simulink model "IntModelY1"  (R2022b)
settings: Solver=VariableStepAuto  StartTime=0.0  StopTime=inf  RelTol=1e-3
model workspace (MAT data in the model file):
  firstWarning = 1
  originalScenarioChecksum = '114339432DE22364D47BB28FC96DC10C'
undefined symbols (not defined in the file): Acceleration, ActorID, AngularVelocity, curvature, curvatureAhd, DefaultGear, DEND_B, DEND_S, DEND_T, direction, driving, gradbp, L, LF, LR, matlabshared, MAX_BRAKE, MAX_STEER, MAX_TORQUE, MCAR, MIN_BRAKE, MIN_STEER, MIN_TORQUE, NUMD_B, NUMD_S, NUMD_T, Pitch, Position, psi_o, R, Roll, RRdamp, SceneInfo, session, sigbuilder_block, STEER_RATIO, stopSign_ID, Tdead, thetaRefs, TL_ID, TrackWidth, Ts, ts, Vdead, Velocity, WB, X_o, xRef2s, Y_o, Yaw, yRef2s
libraries: drivingscenarioandsensors x8, simulink x4, drivingvehiclecontroller x2, trackingutilitieslib x2, simulink_extras x2, robotalgslib x1, mpcadaslib x1, drivinglib x1, autolibshared x1, vehdynlibviscommon x1, vehdynlibsteering x1
(part 1 of 3)
settings Model: Creator=akshran  LastModifiedBy=deepikagiridhar
settings DataIOCC: SignalLogging=off
settings DebuggingCC: UnconnectedInputMsg=warning  UnconnectedOutputMsg=warning  UnconnectedLineMsg=warning
settings ModelReferenceCC: EnableRefExpFcnMdlSchedulingChecks=on
settings RTWCC: DLArmComputeVersion=19.05

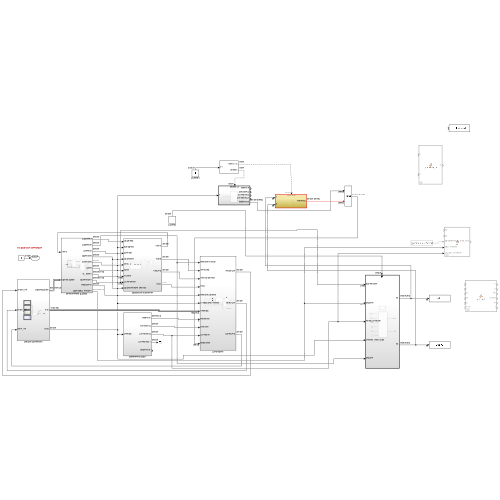
[thumbnail: Simulink's stored preview of the top-level diagram]
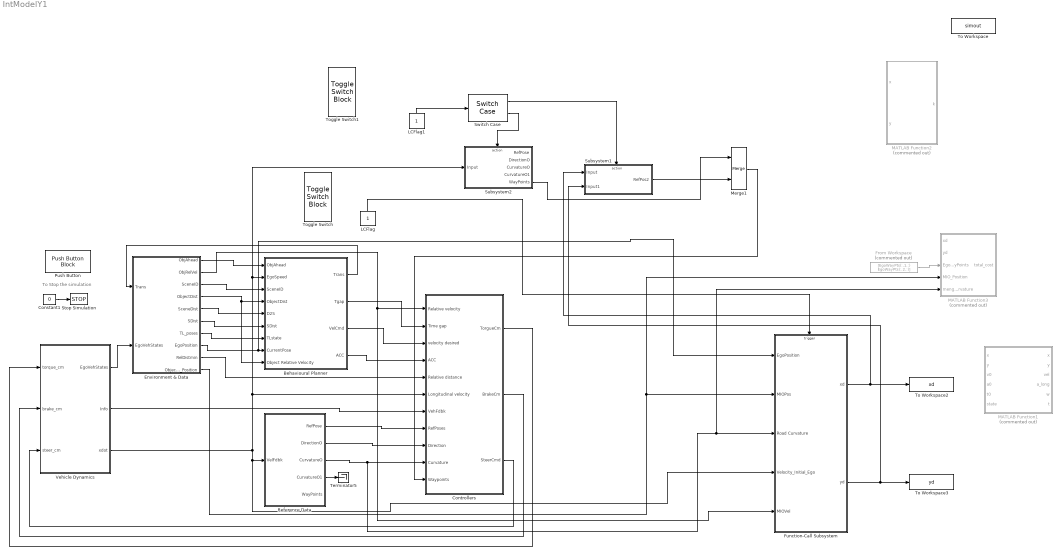
== system IntModelY1 ==
  note: To Stop the simulation
  Behavioural Planner : Subsystem
  Constant1 : Constant  Value=0
  Controllers : Subsystem
  Environment & Data : Subsystem
  From Workspace : FromWorkspace  Commented=on  VariableName=[EgoWayPts(:,1,:) EgoWayPts(:,2,:)]
  Function-Call Subsystem : Subsystem  TreatAsAtomicUnit=on
  LCFlag : Constant
  LCFlag1 : Constant
  MATLAB Function1 : MATLAB Function  Commented=on  TreatAsAtomicUnit=on
  MATLAB Function2 : MATLAB Function  Commented=on  TreatAsAtomicUnit=on
  MATLAB Function3 : MATLAB Function  Commented=on  TreatAsAtomicUnit=on
  Merge1 : Merge
  Push Button : PushButtonBlock  OffValue=1.000000
  Reference Data : Subsystem  VariantControl=Stanley
  Stop Simulation : Stop
  Subsystem1 : Subsystem
  Subsystem2 : Subsystem
  Switch Case : SwitchCase
  Terminator5 : Terminator
  To Workspace : ToWorkspace  VariableName=simout  SaveFormat=Timeseries  SampleTime=-1
  To Workspace2 : ToWorkspace  VariableName=xd  SaveFormat=Timeseries  SampleTime=-1
  To Workspace3 : ToWorkspace  VariableName=yd  SaveFormat=Timeseries  SampleTime=-1
  Toggle Switch : ToggleSwitchBlock
      settings: Values={{'Off', 'On'}, [0 1]}
  Toggle Switch1 : ToggleSwitchBlock
      settings: Values={{'Off', 'On'}, [0 1]}
  Vehicle Dynamics : Subsystem
  wires:
  Environment & Data/4(ObjectDist) -> Behavioural Planner/9(Object Relative Velocity), Behavioural Planner/4(ObjectDist)
  Environment & Data/2(ObjRelVel) -> Function-Call Subsystem/5(MIOVel), Controllers/1(Relative velocity)
  Environment & Data/8(EgoPosition) -> Function-Call Subsystem/1(EgoPosition), Behavioural Planner/8(CurrentPose)
  Vehicle Dynamics/1(EgoVehStates) -> Environment & Data/2(EgoVehStates)
  Vehicle Dynamics/2(Info) -> Controllers/7(VehFdbk)
  Environment & Data/5(SceneDist) -> Behavioural Planner/5(D2S)
  Environment & Data/3(SceneID) -> Behavioural Planner/3(SceneID)
  Behavioural Planner/4(ACC) -> Controllers/4(ACC)
  Environment & Data/9(RelDistmin) -> Controllers/5(Relative distance)
  Environment & Data/1(ObjAhead) -> Behavioural Planner/1(ObjAhead)
  Vehicle Dynamics/3(xdot) -> Subsystem2/1(Input), Behavioural Planner/2(EgoSpeed), Controllers/6(Longitudinal velocity), Function-Call Subsystem/4(Velocity_Initial_Ego), Reference Data/1(VelFdbk)
  Environment & Data/6(SDist) -> Behavioural Planner/6(SDist)
  Environment & Data/7(TL_poses) -> Behavioural Planner/7(TLstate)
  Controllers/2(BrakeCm) -> Vehicle Dynamics/2(brake_cm)
  Behavioural Planner/1(Trans) -> Environment & Data/1(Trans)
  Behavioural Planner/2(Tgap) -> Controllers/2(Time gap)
  Behavioural Planner/3(VelCmd) -> Controllers/3(velocity desired)
  Reference Data/2(DirectionO) -> Controllers/9(Direction)
  Reference Data/3(CurvatureO) -> Function-Call Subsystem/3(Road Curvature), MATLAB Function3/5(menger_curvature), Controllers/10(Curvature)
  Reference Data/4(CurvatureO1) -> Terminator5/1
  Controllers/1(TorgueCm) -> Vehicle Dynamics/1(torque_cm)
  Controllers/3(SteerCmd) -> Vehicle Dynamics/3(steer_cm)
  Constant1/1 -> Stop Simulation/1
  From Workspace/1 -> MATLAB Function3/3(EgoWayPoints)
  Environment & Data/10(ObjectMIO_Position) -> MATLAB Function3/4(MIO_Position), Function-Call Subsystem/2(MIOPos)
  LCFlag/1 -> Function-Call Subsystem/Trigger
  Function-Call Subsystem/1(xd) -> Subsystem1/1(Input), To Workspace2/1
  Function-Call Subsystem/2(yd) -> Subsystem1/2(Input1), To Workspace3/1
  Switch Case/2 -> Subsystem2/Action
  Switch Case/1 -> Subsystem1/Action
  Reference Data/1(RefPose) -> Controllers/8(RefPoses)
  Subsystem2/5(WayPoints) -> Merge1/1
  Merge1/1 -> Controllers/11(Waypoints)
  LCFlag1/1 -> Switch Case/1
  Subsystem1/1(RefPos2) -> Merge1/2

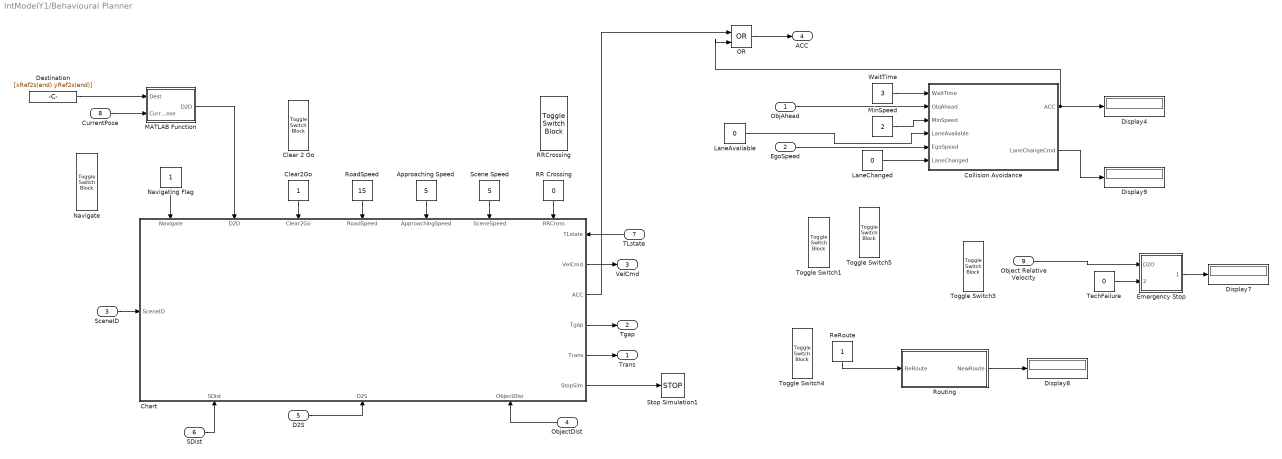
== system IntModelY1/Behavioural Planner ==
  ObjAhead : Inport
  EgoSpeed : Inport  Port=2
  SceneID : Inport  Port=3
  ObjectDist : Inport  Port=4
  D2S : Inport  Port=5
  SDist : Inport  Port=6
  TLstate : Inport  Port=7
  CurrentPose : Inport  Port=8
  Object Relative Velocity : Inport  Port=9
  Approaching Speed : Constant  Value=5
  Chart : Stateflow chart  TreatAsAtomicUnit=on
      settings: PortSchema="{\"entries\":[{\"content\":{\"sides\":[{\"content\":{\"connectorIds\":[\"In12\"]},\"type\":\"ConnectorPlacement.EquallySpacedRectSide\",\"uuid\":\"81aca70f-0947-49fb-b60a-be241e44193b\"},{\"content\":{\"connectorIds\":[\"In1\",\"Out1\",\"Out2\",\"Out3\",\"Out4\",\"Out5\"],\"side\":\"RIGHT\"},\"type\":\"ConnectorPlacement.EquallySpacedRectSide\",\"uuid\":\"e7b9645e-3711-4964-ac9b-0199dd335e99\"},{\"content\":{\"connectorIds\":[\"In8\",\"In9\",\"In10\",\"In11\",\"In2\",\"In4\",\"In6\"],\"side\":\"TOP\"},\"type\":\"ConnectorPlacement.EquallySpacedRectSide\",\"uuid\":\"6876f024-944b-4540-9404-d68f37763657\"},{\"content\":{\"connectorIds\":[\"In5\",\"In7\",\"In3\"],\"side\":\"BOTTOM\"},\"type\":\"ConnectorPlacement.EquallySpacedRectSide\",\"uuid\":\"44acab73-cdde-4edf-95df-27422644ccab\"}]},\"type\":\"ConnectorPlacement.EquallySpacedConnector\",\"uuid\":\"d2c31c01-e447-43db-8d2b-8b98a0ca291a\"}],\"packageUris\":[\"http://schema.mathworks.com/mf0/Connector/R2020b\"],\"version\":\"1.0\"}"
  Clear 2 Go : ToggleSwitchBlock
      settings: Values={{'Off', 'On'}, [0 1]}
  Clear2Go : Constant
  Collision Avoidance : Stateflow chart  TreatAsAtomicUnit=on
  Destination : Constant  Value=[xRef2s(end) yRef2s(end)]
  Display{4,7..9} (4 alike) : Display
  Emergency Stop : Stateflow chart  TreatAsAtomicUnit=on
  LaneAvailable : Constant  Value=0
  LaneChanged : Constant  Value=0
  MATLAB Function : MATLAB Function  TreatAsAtomicUnit=on
  MinSpeed : Constant  Value=2
  Navigate : ToggleSwitchBlock
      settings: Values={{'Off', 'On'}, [0 1]}
  Navigating Flag : Constant
  OR : Logic  Operator=OR  IconShape=distinctive  AllPortsSameDT=off  OutDataTypeStr=fixdt(1,16)
  RR Crossing : Constant  Value=0
  RRCrossing : ToggleSwitchBlock
      settings: Values={{'Off', 'On'}, [0 1]}
  ReRoute : Constant
  RoadSpeed : Constant  Value=15
  Routing : Stateflow chart  TreatAsAtomicUnit=on
  Scene Speed : Constant  Value=5
  Stop Simulation1 : Stop
  TechFailure : Constant  Value=0
  Toggle Switch{1,3..5} (4 alike) : ToggleSwitchBlock
      settings: Values={{'Off', 'On'}, [0 1]}
  WaitTime : Constant  Value=3
  Trans : Outport
  Tgap : Outport  Port=2
  VelCmd : Outport  Port=3
  ACC : Outport  Port=4
  wires:
  Clear2Go/1 -> Chart/10(Clear2Go)
  Routing/1(NewRoute) -> Display8/1
  ObjectDist/1 -> Chart/3(ObjectDist)
  WaitTime/1 -> Collision Avoidance/1(WaitTime)
  Navigating Flag/1 -> Chart/8(Navigate)
  Approaching Speed/1 -> Chart/2(ApproachingSpeed)
  Scene Speed/1 -> Chart/4(SceneSpeed)
  EgoSpeed/1 -> Collision Avoidance/5(EgoSpeed)
  ReRoute/1 -> Routing/1(ReRoute)
  Collision Avoidance/2(LaneChangeCmd) -> Display9/1
  LaneAvailable/1 -> Collision Avoidance/4(LaneAvailable)
  CurrentPose/1 -> MATLAB Function/2(CurrentPose)
  RR Crossing/1 -> Chart/6(RRCross)
  MinSpeed/1 -> Collision Avoidance/3(MinSpeed)
  LaneChanged/1 -> Collision Avoidance/6(LaneChanged)
  RoadSpeed/1 -> Chart/11(RoadSpeed)
  ObjAhead/1 -> Collision Avoidance/2(ObjAhead)
  Destination/1 -> MATLAB Function/1(Dest)
  SceneID/1 -> Chart/12(SceneID)
  MATLAB Function/1(D2D) -> Chart/9(D2D)
  Chart/5(StopSim) -> Stop Simulation1/1
  Chart/4(Trans) -> Trans/1
  TLstate/1 -> Chart/1(TLstate)
  Chart/1(VelCmd) -> VelCmd/1
  SDist/1 -> Chart/5(SDist)
  D2S/1 -> Chart/7(D2S)
  Chart/3(Tgap) -> Tgap/1
  TechFailure/1 -> Emergency Stop/2(TechFailure)
  Emergency Stop/1(EStop) -> Display7/1
  Object Relative Velocity/1 -> Emergency Stop/1(D2O)
  Collision Avoidance/1(ACC) -> OR/2, Display4/1
  OR/1 -> ACC/1
  Chart/2(ACC) -> OR/1

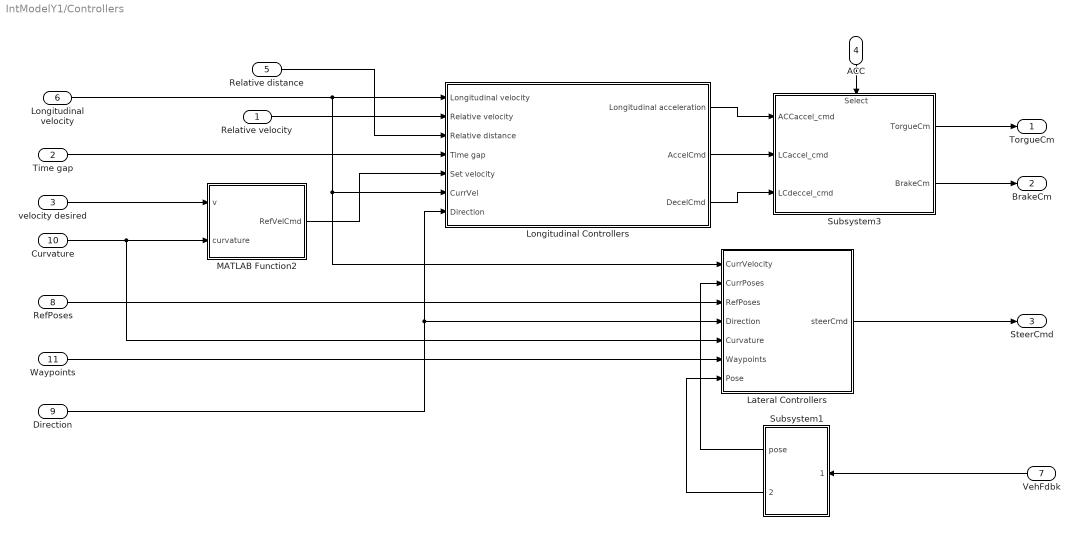
== system IntModelY1/Controllers ==
  Relative velocity : Inport
  Time gap : Inport  Port=2
  velocity desired : Inport  Port=3
  ACC : Inport  Port=4
  Relative distance : Inport  Port=5
  Longitudinal velocity : Inport  Port=6
  VehFdbk : Inport  Port=7
  RefPoses : Inport  Port=8
  Direction : Inport  Port=9
  Curvature : Inport  Port=10
  Waypoints : Inport  Port=11
  Lateral Controllers : Subsystem
  Longitudinal Controllers : Subsystem
  MATLAB Function2 : MATLAB Function  TreatAsAtomicUnit=on
  Subsystem1 : Subsystem
  Subsystem3 : Subsystem
      settings: PortSchema="{\"entries\":[{\"content\":{\"sides\":[{\"content\":{\"connectorIds\":[\"In1\",\"In2\",\"In3\"]},\"type\":\"ConnectorPlacement.EquallySpacedRectSide\",\"uuid\":\"a23b1a10-3bcb-40a0-900c-c9a3f160b173\"},{\"content\":{\"connectorIds\":[\"Out1\",\"Out2\"],\"side\":\"RIGHT\"},\"type\":\"ConnectorPlacement.EquallySpacedRectSide\",\"uuid\":\"88840b66-912f-4184-aeec-297642319416\"},{\"content\":{\"connectorIds\":[\"In4\"],\"side\":\"TOP\"},\"type\":\"ConnectorPlacement.EquallySpacedRectSide\",\"uuid\":\"37a03ca9-b065-473e-b290-3b07703c6005\"}]},\"type\":\"ConnectorPlacement.EquallySpacedConnector\",\"uuid\":\"5bfc7c71-8f7a-4cba-a168-7eeca22a2fcb\"}],\"packageUris\":[\"http://schema.mathworks.com/mf0/Connector/R2020b\"],\"version\":\"1.0\"}"
  TorgueCm : Outport
  BrakeCm : Outport  Port=2
  SteerCmd : Outport  Port=3
  wires:
  Subsystem1/1(pose) -> Lateral Controllers/2(CurrPoses)
  Longitudinal Controllers/1(Longitudinal acceleration) -> Subsystem3/1(ACCaccel_cmd)
  Curvature/1 -> Lateral Controllers/5(Curvature), MATLAB Function2/2(curvature)
  Relative velocity/1 -> Longitudinal Controllers/2(Relative velocity)
  Subsystem1/2(PPpose) -> Lateral Controllers/7(Pose)
  MATLAB Function2/1(RefVelCmd) -> Longitudinal Controllers/5(Set velocity)
  Direction/1 -> Lateral Controllers/4(Direction), Longitudinal Controllers/7(Direction)
  RefPoses/1 -> Lateral Controllers/3(RefPoses)
  velocity desired/1 -> MATLAB Function2/1(v)
  Subsystem3/2(BrakeCm) -> BrakeCm/1
  Longitudinal Controllers/2(AccelCmd) -> Subsystem3/2(LCaccel_cmd)
  Longitudinal Controllers/3(DecelCmd) -> Subsystem3/3(LCdeccel_cmd)
  Longitudinal velocity/1 -> Lateral Controllers/1(CurrVelocity), Longitudinal Controllers/6(CurrVel), Longitudinal Controllers/1(Longitudinal velocity)
  Time gap/1 -> Longitudinal Controllers/4(Time gap)
  Waypoints/1 -> Lateral Controllers/6(Waypoints)
  VehFdbk/1 -> Subsystem1/1(VehFdbk)
  Subsystem3/1(TorgueCm) -> TorgueCm/1
  Lateral Controllers/1(steerCmd) -> SteerCmd/1
  Relative distance/1 -> Longitudinal Controllers/3(Relative distance)
  ACC/1 -> Subsystem3/4(Select)

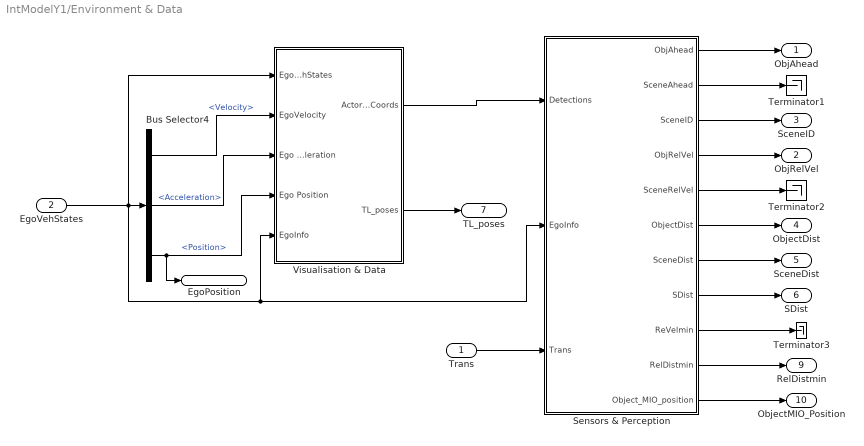
== system IntModelY1/Environment & Data ==
  Trans : Inport
  EgoVehStates : Inport  Port=2
  Bus Selector4 : BusSelector  OutputSignals=Velocity,Acceleration,Position
  Sensors & Perception : Subsystem
  Terminator1 : Terminator
  Terminator2 : Terminator
  Terminator3 : Terminator
  Visualisation & Data : Subsystem
  ObjAhead : Outport
  ObjRelVel : Outport  Port=2
  SceneID : Outport  Port=3
  ObjectDist : Outport  Port=4
  SceneDist : Outport  Port=5
  SDist : Outport  Port=6
  TL_poses : Outport  Port=7
  EgoPosition : Outport  Port=8
  RelDistmin : Outport  Port=9
  ObjectMIO_Position : Outport  Port=10
  wires:
  EgoVehStates/1 -> Visualisation & Data/1(EgoVehStates), Sensors & Perception/2(EgoInfo), Visualisation & Data/5(EgoInfo), Bus Selector4/1
  Bus Selector4/2 -> Visualisation & Data/3(Ego Acceleration)  "<Acceleration>"
  Bus Selector4/1 -> Visualisation & Data/2(EgoVelocity)  "<Velocity>"
  Visualisation & Data/2(TL_poses) -> TL_poses/1
  Sensors & Perception/1(ObjAhead) -> ObjAhead/1
  Sensors & Perception/7(SceneDist) -> SceneDist/1
  Bus Selector4/3 -> Visualisation & Data/4(Ego Position), EgoPosition/1  "<Position>"
  Visualisation & Data/1(Actors_VehCoords) -> Sensors & Perception/1(Detections)
  Trans/1 -> Sensors & Perception/3(Trans)
  Sensors & Perception/2(SceneAhead) -> Terminator1/1
  Sensors & Perception/3(SceneID) -> SceneID/1
  Sensors & Perception/4(ObjRelVel) -> ObjRelVel/1
  Sensors & Perception/5(SceneRelVel) -> Terminator2/1
  Sensors & Perception/6(ObjectDist) -> ObjectDist/1
  Sensors & Perception/8(SDist) -> SDist/1
  Sensors & Perception/9(ReVelmin) -> Terminator3/1
  Sensors & Perception/10(RelDistmin) -> RelDistmin/1
  Sensors & Perception/11(Object_MIO_position) -> ObjectMIO_Position/1

== system IntModelY1/Function-Call Subsystem ==
  EgoPosition : Inport
  MIOPos : Inport  Port=2
  Road Curvature : Inport  Port=3
  Velocity_Initial_Ego : Inport  Port=4
  MIOVel : Inport  Port=5
  function : TriggerPort  VariantControl=(inherit)  ShowOutputPort=on
  Constant : Constant
  MATLAB Function : MATLAB Function  TreatAsAtomicUnit=on
  xd : Outport
  yd : Outport  Port=2
  wires:
  EgoPosition/1 -> MATLAB Function/1(EgoPosition)
  MIOPos/1 -> MATLAB Function/2(MIOPos)
  Road Curvature/1 -> MATLAB Function/3(curvature)
  MIOVel/1 -> MATLAB Function/4(MIOVel)
  Velocity_Initial_Ego/1 -> MATLAB Function/5(V_i)
  MATLAB Function/1(xd) -> xd/1
  MATLAB Function/2(yd) -> yd/1
  Constant/1 -> MATLAB Function/6(lane_side)

== system IntModelY1/Reference Data ==
  note: Select method to calculate theta
  VelFdbk : Inport
  Curvature : Lookup_n-D  NumberOfTableDimensions=1  BreakpointsForDimension1=gradbp  Table=curvature  InternalRulePriority=Speed  RndMeth=Simplest
  CurvatureAhd : Lookup_n-D  Commented=on  NumberOfTableDimensions=1  BreakpointsForDimension1=gradbp  Table=curvatureAhd  InternalRulePriority=Speed  RndMeth=Simplest
  Direction : Lookup_n-D  NumberOfTableDimensions=1  BreakpointsForDimension1=gradbp  Table=direction  InternalRulePriority=Speed  RndMeth=Simplest
  Integrator : Integrator
  Matrix Concatenate : Concatenate  Mode=Multidimensional array  ConcatenateDimension=2
  Mux : Mux  Inputs=3
  Theta : Subsystem  Variant=on  VariantControlMode=label  LabelModeActiveChoice=thetaLookUpTable
  X Ref : Lookup_n-D  NumberOfTableDimensions=1  BreakpointsForDimension1=gradbp  Table=xRef2s  InternalRulePriority=Speed  RndMeth=Simplest
  Y Ref : Lookup_n-D  NumberOfTableDimensions=1  BreakpointsForDimension1=gradbp  Table=yRef2s  InternalRulePriority=Speed  RndMeth=Simplest
  RefPose : Outport
  DirectionO : Outport  Port=2
  CurvatureO : Outport  Port=3
  CurvatureO1 : Outport  Port=4
  WayPoints : Outport  Port=5
  wires:
  Direction/1 -> DirectionO/1
  Curvature/1 -> CurvatureO/1
  Mux/1 -> RefPose/1
  Integrator/1 -> CurvatureAhd/1, Curvature/1, Direction/1, Matrix Concatenate/1, Theta/3(dis), Y Ref/1, Matrix Concatenate/2, X Ref/1
  VelFdbk/1 -> Integrator/1
  Theta/1(theta) -> Mux/3
  CurvatureAhd/1 -> CurvatureO1/1
  Matrix Concatenate/1 -> WayPoints/1
  X Ref/1 -> Theta/2(x), Mux/1
  Y Ref/1 -> Theta/1(y), Mux/2

== system IntModelY1/Subsystem1 ==
  Input : Inport
  Input1 : Inport  Port=2
  Action Port : ActionPort  ActionPortLabel=case [ 1 ]:
  From Workspace : FromWorkspace  Commented=on  VariableName=xRef2
  From Workspace1 : FromWorkspace  Commented=on  VariableName=yRef2
  Matrix Concatenate : Concatenate  Mode=Multidimensional array  ConcatenateDimension=2
  RefPos2 : Outport
  wires:
  Matrix Concatenate/1 -> RefPos2/1
  Input/1 -> Matrix Concatenate/1
  Input1/1 -> Matrix Concatenate/2

== system IntModelY1/Subsystem2 ==
  Input : Inport
  Action Port : ActionPort  ActionPortLabel=default:
  Reference Data : Subsystem  VariantControl=Stanley
  RefPose : Outport
  DirectionO : Outport  Port=2
  CurvatureO : Outport  Port=3
  CurvatureO1 : Outport  Port=4
  WayPoints : Outport  Port=5
  wires:
  Input/1 -> Reference Data/1(VelFdbk)
  Reference Data/1(RefPose) -> RefPose/1
  Reference Data/5(WayPoints) -> WayPoints/1
  Reference Data/4(CurvatureO1) -> CurvatureO1/1
  Reference Data/3(CurvatureO) -> CurvatureO/1
  Reference Data/2(DirectionO) -> DirectionO/1

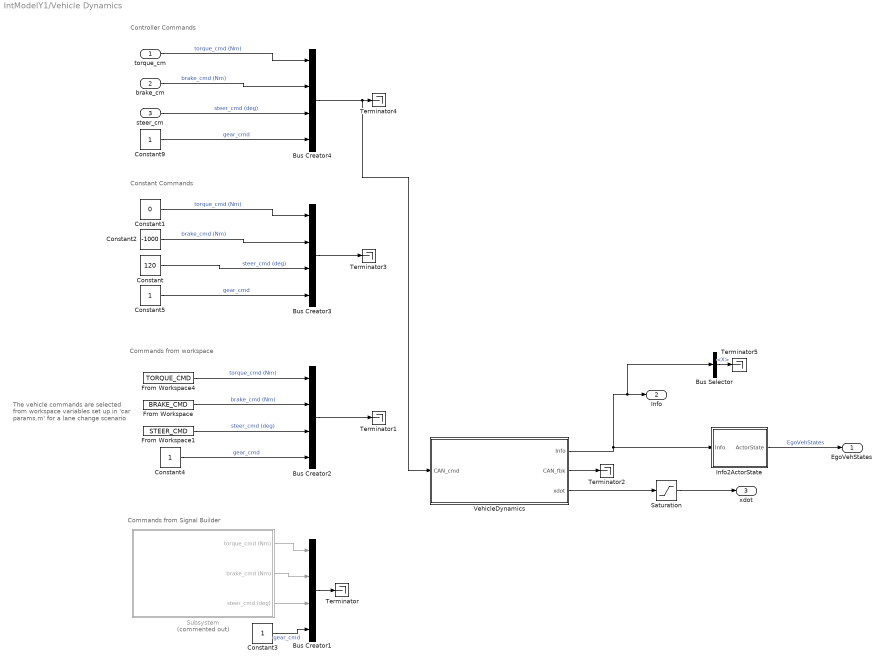
== system IntModelY1/Vehicle Dynamics ==
  note: Constant Commands
  note: Commands from workspace
  note: Commands from Signal Builder
  note: The vehicle commands are selected from workspace variables set up in 'car params.m' for a lane change scenario
  note: Controller Commands
  torque_cm : Inport
  brake_cm : Inport  Port=2
  steer_cm : Inport  Port=3
  Bus Creator{1..4} (4 alike) : BusCreator  Inputs=4
  Bus Selector : BusSelector  OutputSignals=InertFrm.Cg.Disp.X
  Constant : Constant  Value=120
  Constant1 : Constant  Value=0
  Constant2 : Constant  Value=-1000
  Constant{3..5,9} (4 alike) : Constant
  From Workspace : FromWorkspace  VariableName=BRAKE_CMD  SampleTime=ts
  From Workspace1 : FromWorkspace  VariableName=STEER_CMD  SampleTime=ts
  From Workspace4 : FromWorkspace  VariableName=TORQUE_CMD  SampleTime=ts
  Info2ActorState : Subsystem
  Saturation : Saturate  UpperLimit=inf  LowerLimit=0.001
  Subsystem : Subsystem  Commented=on
  Terminator{,1..5} (6 alike) : Terminator
  VehicleDynamics : Subsystem  mask{InitPosition=[X_o Y_o 0], InitSpeed=0, InitYaw=psi_o}
      mask prompts: InitPosition "Initial Position (m)"; InitSpeed "Initial Speed (m/s)"; InitYaw "Init Yaw (rad)"
  EgoVehStates : Outport
  Info : Outport  Port=2
  xdot : Outport  Port=3
  wires:
  Bus Creator2/1 -> Terminator1/1
  VehicleDynamics/2(CAN_fbk) -> Terminator2/1
  VehicleDynamics/1(Info) -> Bus Selector/1, Info/1, Info2ActorState/1(Info)
  Constant/1 -> Bus Creator3/3  "steer_cmd (deg)"
  Info2ActorState/1(ActorState) -> EgoVehStates/1  "EgoVehStates"
  Constant1/1 -> Bus Creator3/1  "torque_cmd (Nm)"
  Constant2/1 -> Bus Creator3/2  "brake_cmd (Nm)"
  VehicleDynamics/3(xdot) -> Saturation/1
  Subsystem/1(torque_cmd (Nm)) -> Bus Creator1/1
  Subsystem/2(brake_cmd (Nm)) -> Bus Creator1/2
  Subsystem/3(steer_cmd (deg)) -> Bus Creator1/3
  Constant3/1 -> Bus Creator1/4  "gear_cmd"
  Constant4/1 -> Bus Creator2/4  "gear_cmd"
  From Workspace/1 -> Bus Creator2/2  "brake_cmd (Nm)"
  From Workspace1/1 -> Bus Creator2/3  "steer_cmd (deg)"
  From Workspace4/1 -> Bus Creator2/1  "torque_cmd (Nm)"
  Constant5/1 -> Bus Creator3/4  "gear_cmd"
  Bus Creator1/1 -> Terminator/1
  brake_cm/1 -> Bus Creator4/2  "brake_cmd (Nm)"
  Constant9/1 -> Bus Creator4/4  "gear_cmd"
  torque_cm/1 -> Bus Creator4/1  "torque_cmd (Nm)"
  steer_cm/1 -> Bus Creator4/3  "steer_cmd (deg)"
  Bus Creator3/1 -> Terminator3/1
  Bus Creator4/1 -> VehicleDynamics/1(CAN_cmd), Terminator4/1
  Saturation/1 -> xdot/1
  Bus Selector/1 -> Terminator5/1  "<X>"

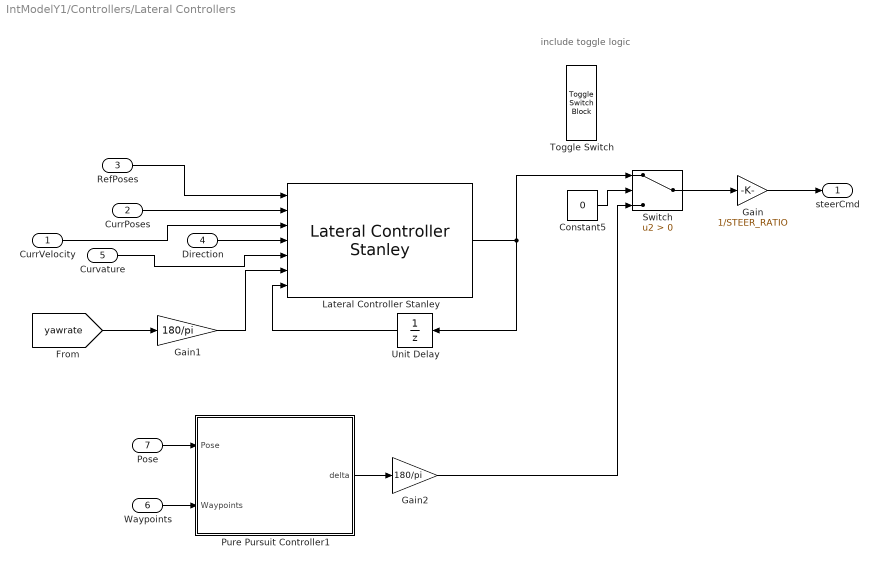
== system IntModelY1/Controllers/Lateral Controllers ==
  note: include toggle logic
  CurrVelocity : Inport
  CurrPoses : Inport  Port=2
  RefPoses : Inport  Port=3
  Direction : Inport  Port=4
  Curvature : Inport  Port=5
  Waypoints : Inport  Port=6
  Pose : Inport  Port=7
  Constant5 : Constant  Value=0
  Gain : Gain  Gain=1/STEER_RATIO
  Gain1 : Gain  Gain=180/pi
  Gain2 : Gain  Gain=180/pi
  Lateral Controller Stanley : drivingvehiclecontroller/Lateral Controller Stanley  ModelType=Dynamic bicycle model  PositionGainF=2.5  PositionGainR=2.5  YawRateGain=0.2  DelayGain=0.2  VehicleMass=MCAR  Lf=LF  Lr=LR  TireStiffness=5e3  Wheelbase=3  MaxSteeringAngle=80
  Pure Pursuit Controller1 : Subsystem
  Switch : Switch  Criteria=u2 > Threshold  SaturateOnIntegerOverflow=off  InputSameDT=off
  Toggle Switch : ToggleSwitchBlock
      settings: Values={{'Off', 'On'}, [0 1]}
  Unit Delay : UnitDelay  SampleTime=-1  HasFrameUpgradeWarning=on
  steerCmd : Outport
  wires:
  Gain2/1 -> Switch/3
  Direction/1 -> Lateral Controller Stanley/4
  [yawrate] -> Gain1/1
  Constant5/1 -> Switch/2
  Lateral Controller Stanley/1 -> Switch/1, Unit Delay/1
  Unit Delay/1 -> Lateral Controller Stanley/7
  Switch/1 -> Gain/1
  CurrPoses/1 -> Lateral Controller Stanley/2
  Gain1/1 -> Lateral Controller Stanley/6
  Pure Pursuit Controller1/1(delta) -> Gain2/1
  Gain/1 -> steerCmd/1
  Curvature/1 -> Lateral Controller Stanley/5
  CurrVelocity/1 -> Lateral Controller Stanley/3
  Waypoints/1 -> Pure Pursuit Controller1/2(Waypoints)
  RefPoses/1 -> Lateral Controller Stanley/1
  Pose/1 -> Pure Pursuit Controller1/1(Pose)

== system IntModelY1/Controllers/Longitudinal Controllers ==
  Longitudinal velocity : Inport
  Relative velocity : Inport  Port=2
  Relative distance : Inport  Port=3
  Time gap : Inport  Port=4
  Set velocity : Inport  Port=5
  CurrVel : Inport  Port=6
  Direction : Inport  Port=7
  Adaptive Cruise Control System : mpcadaslib/Adaptive Cruise Control System  EgoModel=tf(1,[0.5,1,0])  InitialEgoVelocity=0  DefaultSpacing=WB+2  MaxVelocity=50  MinAcceleration=-40  amin_ext=off  MaxAcceleration=40  amax_ext=off  Ts=0.1  PredictionHorizon=10  ControllerBehavior=1.0  suboptimal=off  maxiter=10  datatypeopt=double  optmode=off  trackmode=off
  Constant3 : Constant  Value=0
  Longitudinal Controller Stanley : drivingvehiclecontroller/Longitudinal Controller Stanley  Kp=10  Ki=0.1  SampleTime=0.05  MaxAcceleration=40  MaxDeceleration=40
  Longitudinal acceleration : Outport
  AccelCmd : Outport  Port=2
  DecelCmd : Outport  Port=3
  wires:
  Set velocity/1 -> Adaptive Cruise Control System/1, Longitudinal Controller Stanley/1
  Constant3/1 -> Longitudinal Controller Stanley/4
  Longitudinal velocity/1 -> Adaptive Cruise Control System/3
  CurrVel/1 -> Longitudinal Controller Stanley/2
  Longitudinal Controller Stanley/1 -> AccelCmd/1
  Longitudinal Controller Stanley/2 -> DecelCmd/1
  Direction/1 -> Longitudinal Controller Stanley/3
  Relative velocity/1 -> Adaptive Cruise Control System/5
  Relative distance/1 -> Adaptive Cruise Control System/4
  Adaptive Cruise Control System/1 -> Longitudinal acceleration/1
  Time gap/1 -> Adaptive Cruise Control System/2

== system IntModelY1/Controllers/Subsystem1 ==
  VehFdbk : Inport
  Bus Selector : BusSelector  OutputSignals=InertFrm.Cg.Disp.X,InertFrm.Cg.Disp.Y,InertFrm.Cg.Ang.psi
  Bus Selector1 : BusSelector  Commented=on  OutputSignals=InertFrm.Cg.Disp.X,InertFrm.Cg.Disp.Y,InertFrm.Cg.Disp.Z
  Gain1 : Gain  Gain=180/pi
  Mux : Mux  Inputs=3
  Mux1 : Mux  Commented=on  Inputs=3
  Mux2 : Mux  Inputs=3
  Transpose : Math  Operator=transpose  SignedPower=on
  Transpose1 : Math  Commented=on  Operator=transpose  SignedPower=on
  Transpose2 : Math  Operator=transpose  SignedPower=on
  pose : Outport
  PPpose : Outport  Port=2
  wires:
  Mux/1 -> Transpose/1
  VehFdbk/1 -> Bus Selector1/1, Bus Selector/1
  Gain1/1 -> Mux/3
  Transpose/1 -> pose/1
  Bus Selector/3 -> Mux2/3, Gain1/1  "<psi>"
  Bus Selector1/1 -> Mux1/1  "<X>"
  Bus Selector1/2 -> Mux1/2  "<Y>"
  Bus Selector1/3 -> Mux1/3  "<Z>"
  Mux1/1 -> Transpose1/1
  Mux2/1 -> Transpose2/1
  Transpose2/1 -> PPpose/1
  Bus Selector/2 -> Mux/2, Mux2/2  "<Y>"
  Bus Selector/1 -> Mux/1, Mux2/1  "<X>"

== system IntModelY1/Controllers/Subsystem3 ==
  ACCaccel_cmd : Inport
  LCaccel_cmd : Inport  Port=2
  LCdeccel_cmd : Inport  Port=3
  Select : Inport  Port=4
  Merge1 : Merge
  Merge2 : Merge
  Subsystem1 : Subsystem
  Subsystem2 : Subsystem
  Switch Case1 : SwitchCase  CaseConditions={1, 0}  ShowDefaultCase=off
  TorgueCm : Outport
  BrakeCm : Outport  Port=2
  wires:
  LCdeccel_cmd/1 -> Subsystem1/2(decc_cmd)
  Subsystem1/2(brake_cm) -> Merge2/2
  Subsystem1/1(torque_cm) -> Merge1/2
  Subsystem2/2(brake_cm) -> Merge2/1
  Switch Case1/1 -> Subsystem2/Action
  Switch Case1/2 -> Subsystem1/Action
  Subsystem2/1(torque_cm) -> Merge1/1
  LCaccel_cmd/1 -> Subsystem1/1(acc_cmd)
  Merge2/1 -> BrakeCm/1
  ACCaccel_cmd/1 -> Subsystem2/1(acc_cmd)
  Merge1/1 -> TorgueCm/1
  Select/1 -> Switch Case1/1

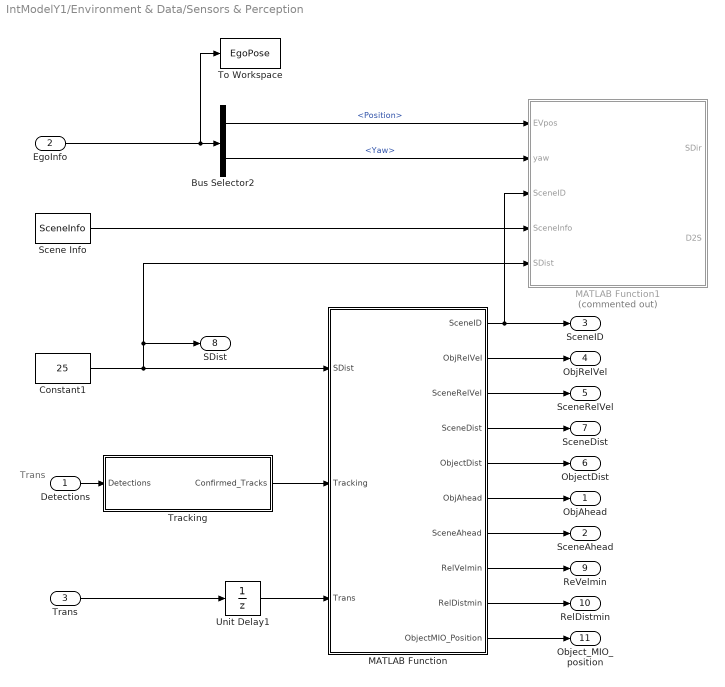
== system IntModelY1/Environment & Data/Sensors & Perception ==
  note: Trans
  Detections : Inport
  EgoInfo : Inport  Port=2
  Trans : Inport  Port=3
  Bus Selector2 : BusSelector  OutputSignals=Position,Yaw
  Constant1 : Constant  Value=25
  MATLAB Function : MATLAB Function  TreatAsAtomicUnit=on
  MATLAB Function1 : MATLAB Function  Commented=on  TreatAsAtomicUnit=on
  Scene Info : Constant  Value=SceneInfo  VectorParams1D=off
  To Workspace : ToWorkspace  VariableName=EgoPose  SaveFormat=Timeseries  SampleTime=-1
  Tracking : Subsystem
  Unit Delay1 : UnitDelay  SampleTime=-1  HasFrameUpgradeWarning=on
  ObjAhead : Outport
  SceneAhead : Outport  Port=2
  SceneID : Outport  Port=3
  ObjRelVel : Outport  Port=4
  SceneRelVel : Outport  Port=5
  ObjectDist : Outport  Port=6
  SceneDist : Outport  Port=7
  SDist : Outport  Port=8
  ReVelmin : Outport  Port=9
  RelDistmin : Outport  Port=10
  Object_MIO_position : Outport  Port=11
  wires:
  MATLAB Function/6(ObjAhead) -> ObjAhead/1
  MATLAB Function/5(ObjectDist) -> ObjectDist/1
  MATLAB Function/7(SceneAhead) -> SceneAhead/1
  MATLAB Function/2(ObjRelVel) -> ObjRelVel/1
  EgoInfo/1 -> To Workspace/1, Bus Selector2/1
  Bus Selector2/1 -> MATLAB Function1/1(EVpos)  "<Position>"
  Detections/1 -> Tracking/1(Detections)
  Scene Info/1 -> MATLAB Function1/4(SceneInfo)
  Bus Selector2/2 -> MATLAB Function1/2(yaw)  "<Yaw>"
  Tracking/1(Confirmed_Tracks) -> MATLAB Function/2(Tracking)
  Constant1/1 -> MATLAB Function1/5(SDist), SDist/1, MATLAB Function/1(SDist)
  MATLAB Function/1(SceneID) -> SceneID/1, MATLAB Function1/3(SceneID)
  MATLAB Function/4(SceneDist) -> SceneDist/1
  MATLAB Function/3(SceneRelVel) -> SceneRelVel/1
  MATLAB Function/8(RelVelmin) -> ReVelmin/1
  MATLAB Function/9(RelDistmin) -> RelDistmin/1
  Trans/1 -> Unit Delay1/1
  Unit Delay1/1 -> MATLAB Function/3(Trans)
  MATLAB Function/10(ObjectMIO_Position) -> Object_MIO_position/1

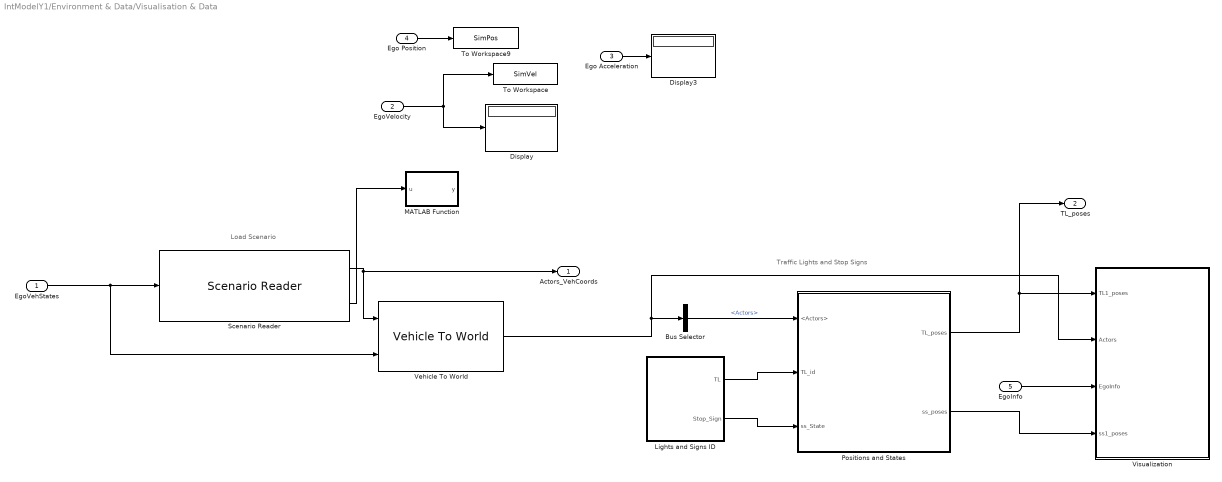
== system IntModelY1/Environment & Data/Visualisation & Data ==
  note: Load Scenario
  note: Traffic Lights and Stop Signs
  EgoVehStates : Inport
  EgoVelocity : Inport  Port=2
  Ego Acceleration : Inport  Port=3
  Ego Position : Inport  Port=4
  EgoInfo : Inport  Port=5
  Bus Selector : BusSelector  OutputSignals=Actors
  Display : Display
  Display3 : Display
  Lights and Signs ID : Subsystem
  MATLAB Function : MATLAB Function  TreatAsAtomicUnit=on
  "Positions and States " : Subsystem
  Scenario Reader : drivingscenarioandsensors/Scenario Reader  ScenarioSource=From file  ScenarioFileName=/Users/deepikagiridhar/Documents/AutoDrive/ADC_Y2/AD_Simulation/planningControl-Simulation/scenarios/highwaylane.mat  ScenarioVariableName=scenario  OutputCoordinateSystem=Vehicle coordinates  EgoVehicleSource=Input port  EgoVehicleActorID=1  OrientVehiclesOnRoad=on  OutputEgoVehiclePose=on  OutputEgoVehicleState=off  SampleTime=Ts  LaneBoundaryOutput=All lane boundaries  LaneBoundaryDistance=0:0.5:9.5  LaneBoundaryLocation=Center of lane markings  BusNameSource=Auto  BusName=BusActors  BusNumActorsSource=Scenario  BusNumActors=100  BusName2Source=Auto  BusName2=BusLaneBoundaries  BusNumLaneBoundariesSource=Scenario  BusNumLaneBoundaries=10  BusName3Source=Auto  BusName3=BusEgoActor  BusName4Source=Auto  BusName4=BusEgoState  ShowCoordinateLabels=on  SimulateUsing=Interpreted execution
  To Workspace : ToWorkspace  VariableName=SimVel  SampleTime=-1
      settings: Save2DSignal=2-D array (concatenate along first dimension)
  To Workspace9 : ToWorkspace  VariableName=SimPos  SampleTime=-1
      settings: Save2DSignal=2-D array (concatenate along first dimension)
  Vehicle To World : drivingscenarioandsensors/Vehicle To World  BusNameSource=Auto  BusName=BusVehicleToWorldActors  SimulateUsing=Interpreted execution
  Visualization : Subsystem
  Actors_VehCoords : Outport
  TL_poses : Outport  Port=2
  wires:
  Vehicle To World/1 -> Visualization/2(Actors), Bus Selector/1
  EgoVelocity/1 -> To Workspace/1, Display/1
  Scenario Reader/1 -> Vehicle To World/1, Actors_VehCoords/1
  "Positions and States "/1(TL_poses) -> TL_poses/1, Visualization/1(TL1_poses)
  Lights and Signs ID/1(TL) -> "Positions and States "/2(TL_id)
  Bus Selector/1 -> "Positions and States "/1(<Actors>)  "<Actors>"
  Lights and Signs ID/2(Stop_Sign) -> "Positions and States "/3(ss_State)
  "Positions and States "/2(ss_poses) -> Visualization/4(ss1_poses)
  Ego Acceleration/1 -> Display3/1
  Ego Position/1 -> To Workspace9/1
  EgoInfo/1 -> Visualization/3(EgoInfo)
  EgoVehStates/1 -> Vehicle To World/2, Scenario Reader/1
  Scenario Reader/2 -> MATLAB Function/1(u)

== system IntModelY1/Reference Data/Theta ==
  note: 1) Add Subsystem or Model blocks as valid variant choices.
      | 2) You cannot connect blocks at this level. At simulation, connectivity is automatically
      | determined, based on the active variant and port name matching.
  y : Inport
  x : Inport  Port=2
  dis : Inport  Port=3
  thetaBlocks : Subsystem  VariantControl=thetaSimulinkBlock
  thetaLt : Subsystem  VariantControl=thetaLookUpTable
  theta : Outport

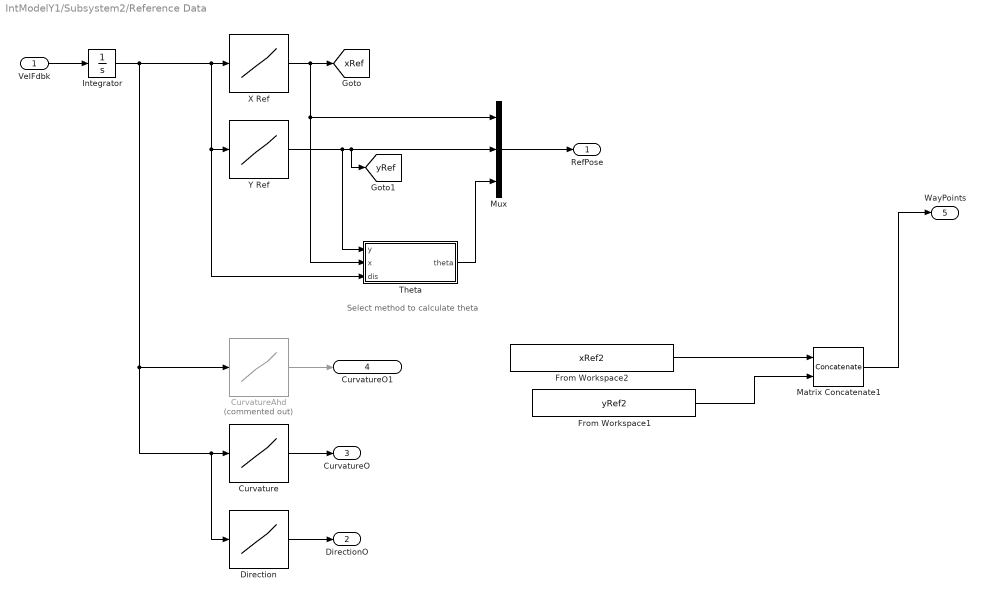
== system IntModelY1/Subsystem2/Reference Data ==
  note: Select method to calculate theta
  VelFdbk : Inport
  Curvature : Lookup_n-D  NumberOfTableDimensions=1  BreakpointsForDimension1=gradbp  Table=curvature  InternalRulePriority=Speed  RndMeth=Simplest
  CurvatureAhd : Lookup_n-D  Commented=on  NumberOfTableDimensions=1  BreakpointsForDimension1=gradbp  Table=curvatureAhd  InternalRulePriority=Speed  RndMeth=Simplest
  Direction : Lookup_n-D  NumberOfTableDimensions=1  BreakpointsForDimension1=gradbp  Table=direction  InternalRulePriority=Speed  RndMeth=Simplest
  From Workspace1 : FromWorkspace  VariableName=yRef2  SampleTime=-1
  From Workspace2 : FromWorkspace  VariableName=xRef2  SampleTime=-1
  Integrator : Integrator
  Matrix Concatenate1 : Concatenate  Mode=Multidimensional array  ConcatenateDimension=2
  Mux : Mux  Inputs=3
  Theta : Subsystem  Variant=on  VariantControlMode=label  LabelModeActiveChoice=thetaLookUpTable
  X Ref : Lookup_n-D  NumberOfTableDimensions=1  BreakpointsForDimension1=gradbp  Table=xRef2s  InternalRulePriority=Speed  RndMeth=Simplest
  Y Ref : Lookup_n-D  NumberOfTableDimensions=1  BreakpointsForDimension1=gradbp  Table=yRef2s  InternalRulePriority=Speed  RndMeth=Simplest
  RefPose : Outport
  DirectionO : Outport  Port=2
  CurvatureO : Outport  Port=3
  CurvatureO1 : Outport  Port=4
  WayPoints : Outport  Port=5
  tag scope: xRef=global, yRef=global
  wires:
  Direction/1 -> DirectionO/1
  Curvature/1 -> CurvatureO/1
  Mux/1 -> RefPose/1
  Integrator/1 -> CurvatureAhd/1, Curvature/1, Direction/1, Theta/3(dis), Y Ref/1, X Ref/1
  VelFdbk/1 -> Integrator/1
  Theta/1(theta) -> Mux/3
  CurvatureAhd/1 -> CurvatureO1/1
  X Ref/1 -> Theta/2(x), Mux/1, [xRef]
  Y Ref/1 -> Theta/1(y), Mux/2, [yRef]
  From Workspace2/1 -> Matrix Concatenate1/1
  From Workspace1/1 -> Matrix Concatenate1/2
  Matrix Concatenate1/1 -> WayPoints/1

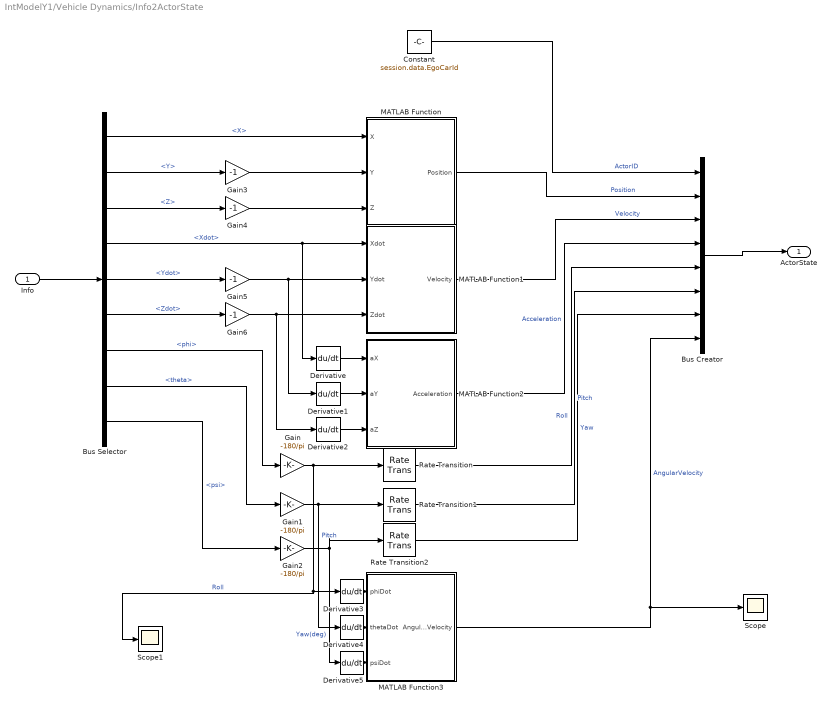
== system IntModelY1/Vehicle Dynamics/Info2ActorState ==
  Info : Inport
  Bus Creator : BusCreator  Inputs=ActorID,Position,Velocity,Acceleration,Roll,Pitch,Yaw,AngularVelocity  OutDataTypeStr=Bus: BusActorState  NonVirtualBus=on
  Bus Selector : BusSelector  OutputSignals=InertFrm.Cg.Disp.X,InertFrm.Cg.Disp.Y,InertFrm.Cg.Disp.Z,InertFrm.Cg.Vel.Xdot,InertFrm.Cg.Vel.Ydot,InertFrm.Cg.Vel.Zdot,InertFrm.Cg.Ang.phi,InertFrm.Cg.Ang.theta,InertFrm.Cg.Ang.psi
  Constant : Constant  Value=session.data.EgoCarId  SampleTime=0.05
  Derivative{,1..5} (6 alike) : Derivative
  Gain : Gain  Gain=-180/pi
  Gain1 : Gain  Gain=-180/pi
  Gain2 : Gain  Gain=-180/pi
  Gain{3..6} (4 alike) : Gain  Gain=-1
  MATLAB Function : MATLAB Function  TreatAsAtomicUnit=on  SystemSampleTime=0.05
  MATLAB Function1 : MATLAB Function  TreatAsAtomicUnit=on  SystemSampleTime=0.05
  MATLAB Function2 : MATLAB Function  TreatAsAtomicUnit=on  SystemSampleTime=0.05
  MATLAB Function3 : MATLAB Function  TreatAsAtomicUnit=on  SystemSampleTime=0.05
  Rate Transition : RateTransition  OutPortSampleTime=0.05
  Rate Transition1 : RateTransition  OutPortSampleTime=0.05
  Rate Transition2 : RateTransition  OutPortSampleTime=0.05
  Scope : Scope
  Scope1 : Scope
  ActorState : Outport
  wires:
  Gain/1 -> Scope1/1, Derivative3/1, Rate Transition/1  "Roll"
  Derivative4/1 -> MATLAB Function3/2(thetaDot)
  Bus Selector/2 -> Gain3/1  "<Y>"
  Bus Selector/4 -> Derivative/1, MATLAB Function1/1(Xdot)  "<Xdot>"
  MATLAB Function1/1(Velocity) -> Bus Creator/3  "Velocity"
  MATLAB Function/1(Position) -> Bus Creator/2  "Position"
  Derivative1/1 -> MATLAB Function2/2(aY)
  Bus Selector/5 -> Gain5/1  "<Ydot>"
  Bus Selector/1 -> MATLAB Function/1(X)  "<X>"
  Bus Selector/9 -> Gain2/1  "<psi>"
  Gain2/1 -> Rate Transition2/1, Derivative5/1  "Yaw(deg)"
  Derivative5/1 -> MATLAB Function3/3(psiDot)
  Bus Selector/7 -> Gain/1  "<phi>"
  MATLAB Function2/1(Acceleration) -> Bus Creator/4  "Acceleration"
  Derivative3/1 -> MATLAB Function3/1(phiDot)
  Gain1/1 -> Derivative4/1, Rate Transition1/1  "Pitch"
  Bus Selector/6 -> Gain6/1  "<Zdot>"
  Bus Selector/8 -> Gain1/1  "<theta>"
  MATLAB Function3/1(AngularVelocity) -> Bus Creator/8, Scope/1  "AngularVelocity"
  Bus Selector/3 -> Gain4/1  "<Z>"
  Derivative2/1 -> MATLAB Function2/3(aZ)
  Derivative/1 -> MATLAB Function2/1(aX)
  Info/1 -> Bus Selector/1
  Constant/1 -> Bus Creator/1  "ActorID"
  Bus Creator/1 -> ActorState/1
  Rate Transition/1 -> Bus Creator/5  "Roll"
  Rate Transition1/1 -> Bus Creator/6  "Pitch"
  Rate Transition2/1 -> Bus Creator/7  "Yaw"
  Gain3/1 -> MATLAB Function/2(Y)
  Gain4/1 -> MATLAB Function/3(Z)
  Gain5/1 -> Derivative1/1, MATLAB Function1/2(Ydot)
  Gain6/1 -> Derivative2/1, MATLAB Function1/3(Zdot)

== system IntModelY1/Vehicle Dynamics/Subsystem ==
  Gain : Gain  Gain=MAX_TORQUE*0.1
  Gain1 : Gain  Gain=MIN_BRAKE*0.06
  Gain2 : Gain  Gain=MAX_STEER/4.5
  Signal Builder : Subsystem  Tag=STV Subsys  LoadFcn=sigbuilder_block('load');  StartFcn=sigbuilder_block('start');  StopFcn=sigbuilder_block('stop');  ClipboardFcn=sigbuilder_block('clipboard');  mask(Sigbuilder block){tuvar=[0:10]}
      mask help: Simulink:masks:SigbuilderBlock_MD
      mask init:
      | if ~strcmp(get_param(bdroot(gcbh),'SimulationStatus'),'stopped') tuvar = sigbuilder_block('maskInit'); end
      settings: CopyFcn=sigbuilder_block('copy');  DeleteFcn=sigbuilder_block('delete');  ModelCloseFcn=sigbuilder_block('modelClose');  PreSaveFcn=sigbuilder_block('preSave');  PauseFcn=sigbuilder_block('pause');  ContinueFcn=sigbuilder_block('continue');  NameChangeFcn=sigbuilder_block('namechange');  OpenFcn=sigbuilder_block('open',[0 30 960 455.5 ]);  CloseFcn=sigbuilder_block('close');
      mask Display: plot(0, 0, 100, 100,[2, 2, 32, 32, 2], [68, 8, 8, 68, 68],[32, 2], [38, 38], [32, 19, 2],[53, 60, 44], [32, 17, 17, 2],[16, 16, 31, 31]);txt = getActiveGroup(gcbh);text(2, 100, txt,'verticalAlignment', 'top');
  torque_cmd (Nm) : Outport
  brake_cmd (Nm) : Outport  Port=2
  steer_cmd (deg) : Outport  Port=3
  wires:
  Gain2/1 -> steer_cmd (deg)/1  "steer_cmd (deg)"
  Signal Builder/1(Normalized Torque) -> Gain/1
  Signal Builder/2(Normalized Brake) -> Gain1/1
  Signal Builder/3(Normalized Steer) -> Gain2/1  "steer_cmd (deg)"
  Gain1/1 -> brake_cmd (Nm)/1  "brake_cmd (Nm)"
  Gain/1 -> torque_cmd (Nm)/1  "torque_cmd (Nm)"

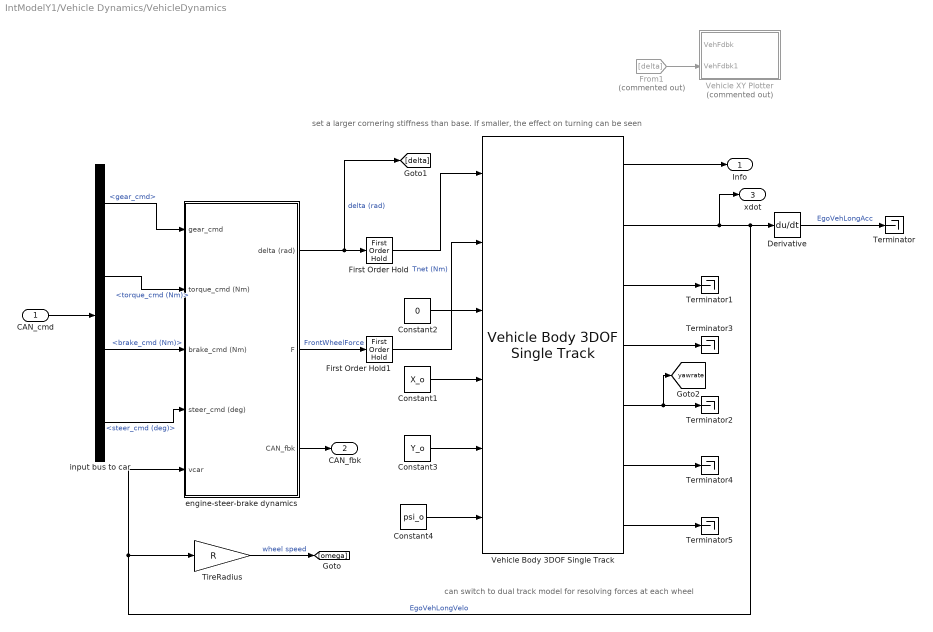
== system IntModelY1/Vehicle Dynamics/VehicleDynamics ==
  note: set a larger cornering stiffness than base. If smaller, the effect on turning can be seen
  note: can switch to dual track model for resolving forces at each wheel
  CAN_cmd : Inport
  Constant1 : Constant  Value=X_o
  Constant2 : Constant  Value=0
  Constant3 : Constant  Value=Y_o
  Constant4 : Constant  Value=psi_o
  Derivative : Derivative
  First Order Hold : FirstOrderHold  ErrorTolerance=inf
  First Order Hold1 : FirstOrderHold  ErrorTolerance=inf
  From1 : From  Commented=on  GotoTag=delta
  Terminator{,1..5} (6 alike) : Terminator
  TireRadius : Gain  Gain=R
  Vehicle Body 3DOF Single Track : autolibshared/Vehicle Body 3DOF Single Track  trackMode=Single (bicycle)  inputMode=External longitudinal forces  frontSteerMode=on  rearSteerMode=off  windMode=off  muMode=off  extFMode=off  extMMode=off  htchFMode=off  htchMMode=off  extXo=on  extpsio=on  extxdoto=off  extro=off  extYo=on  extTamb=off  extydoto=off  aMode=2  NF=2  NR=2  m=MCAR  a=LF  b=LR  h=0.35  dh=1  hh=0.2  X_o=InitPosition(1)  xdot_o=InitSpeed  CalphaMode=off  sigmaMode=on  d=0  hl=0  w=[1.4,1.4]  Cy_f=12e3*100  Cy_r=11e3*100  sigma_f=.1  sigma_r=.1  alpha_f_brk=[-.1 .1]  Cy_f_data=[-9e3 9e3]  alpha_r_brk=[-.1 .1]  Cy_r_data=[-9e3 9e3]  Y_o=-InitPosition(2)  ydot_o=0  Izz=2050  psi_o=-InitYaw/180*pi  r_o=0  Af=2  Cd=.3  Cl=.1  Cpm=.1  beta_w=[0:0.01:0.3]  Cs=[0:0.03:0.9]  Cym=[0:0.01:0.3]  Pabs=101325  Tair=273  g=9.81  mu=1  xdot_tol=.01  Fznom=5000  Fxtire_sat=7e4  Fytire_sat=7e4  longOff=0  latOff=0  vertOff=0  wrapAng=off
  Vehicle XY Plotter : Subsystem  Commented=on  mask(Vehicle XY Plotter){a=LF, b=LR, w=TrackWidth, bufferSize=1024, pltDT=.1}
      mask prompts: a "Distance to front axle from CG, a [m]:"; b "Distance to rear axle from CG, b [m]:"; w "Track width, w [m]:"; bufferSize "Path buffer sampe size, bufferSize []:"; pltDT "Plot update rate, pltDT [s]:"
      mask help: This block will display a MATLAB figure which indicates the vehicle path, current position and heading velocity.
      mask TypeOptions a: Vehicle XY Plotter/a
      mask TypeOptions b: Vehicle XY Plotter/b
      mask TypeOptions w: Vehicle XY Plotter/w
      mask TypeOptions bufferSize: Vehicle XY Plotter/bufferSize
  engine-steer-brake dynamics : Subsystem
  input bus to car : BusSelector  OutputSignals=gear_cmd,torque_cmd (Nm),brake_cmd (Nm),steer_cmd (deg)
  Info : Outport
  CAN_fbk : Outport  Port=2  VectorParamsAs1DForOutWhenUnconnected=off
  xdot : Outport  Port=3
  tag scope: yawrate=global
  wires:
  TireRadius/1 -> [omega]  "wheel speed"
  Vehicle Body 3DOF Single Track/1 -> Info/1
  From1/1 -> Vehicle XY Plotter/2(VehFdbk1)
  input bus to car/1 -> engine-steer-brake dynamics/1(gear_cmd)  "<gear_cmd>"
  input bus to car/3 -> engine-steer-brake dynamics/3(brake_cmd (Nm))  "<brake_cmd (Nm)>"
  engine-steer-brake dynamics/1(delta (rad)) -> [delta], First Order Hold/1  "delta (rad)"
  input bus to car/2 -> engine-steer-brake dynamics/2(torque_cmd (Nm))  "<torque_cmd (Nm)>"
  input bus to car/4 -> engine-steer-brake dynamics/4(steer_cmd (deg))  "<steer_cmd (deg)>"
  engine-steer-brake dynamics/3(CAN_fbk) -> CAN_fbk/1
  CAN_cmd/1 -> input bus to car/1
  Constant2/1 -> Vehicle Body 3DOF Single Track/3
  engine-steer-brake dynamics/2(F) -> First Order Hold1/1  "FrontWheelForce"
  First Order Hold/1 -> Vehicle Body 3DOF Single Track/1
  Vehicle Body 3DOF Single Track/2 -> xdot/1, engine-steer-brake dynamics/5(vcar), TireRadius/1, Derivative/1  "EgoVehLongVelo"
  Vehicle Body 3DOF Single Track/3 -> Terminator1/1
  Vehicle Body 3DOF Single Track/4 -> Terminator3/1
  Vehicle Body 3DOF Single Track/5 -> [yawrate], Terminator2/1
  Vehicle Body 3DOF Single Track/6 -> Terminator4/1
  Vehicle Body 3DOF Single Track/7 -> Terminator5/1
  Derivative/1 -> Terminator/1  "EgoVehLongAcc"
  First Order Hold1/1 -> Vehicle Body 3DOF Single Track/2  "Tnet (Nm)"
  Constant1/1 -> Vehicle Body 3DOF Single Track/4
  Constant3/1 -> Vehicle Body 3DOF Single Track/5
  Constant4/1 -> Vehicle Body 3DOF Single Track/6

== system IntModelY1/Controllers/Lateral Controllers/Pure Pursuit Controller1 ==
  note: The subsystem implements a Pure Pursuit controller. The "Pure Pursuit" block calculates the target direction and the "Wheel Steering Angle Formulation" block calculates the wheel steering angle.
  Pose : Inport
  Waypoints : Inport  Port=2
  Pure Pursuit : robotalgslib/Pure Pursuit  DesiredLinearVelocity=1  MaxAngularVelocity=1.0  LookaheadDistance=10  TargetDirPort=on  SimulateUsing=Code generation
  Terminator6 : Terminator
  Terminator7 : Terminator
  Wheel Steering Angle Formulation : Subsystem  mask{L=L, ld=10}
      mask prompts: L "Bicycle length"; ld "Lookahead distance"
      mask TypeOptions L: Bicycle length/Value
      mask TypeOptions ld: Lookahead distance/Value
      mask Display:
      | image("GeometryMask.png")
      | port_label('input', 1, 'alpha')
      | port_label('output', 1, 'delta')
  delta : Outport
  wires:
  Wheel Steering Angle Formulation/1(Al) -> delta/1
  Pure Pursuit/3 -> Wheel Steering Angle Formulation/1(alpha)
  Pure Pursuit/2 -> Terminator7/1
  Pose/1 -> Pure Pursuit/1
  Pure Pursuit/1 -> Terminator6/1
  Waypoints/1 -> Pure Pursuit/2

== system IntModelY1/Controllers/Subsystem3/Subsystem1 ==
  acc_cmd : Inport
  decc_cmd : Inport  Port=2
  Action Port : ActionPort  ActionPortLabel=case [ 0 ]:
  Brake Saturation : Saturate  UpperLimit=MAX_BRAKE  LowerLimit=MIN_BRAKE
  Constant : Constant  Value=0
  Subsystem2 : Subsystem
  Switch : Switch  Criteria=u2 > Threshold  Threshold=500  SaturateOnIntegerOverflow=off  InputSameDT=off
  Switch1 : Switch  Criteria=u2 > Threshold  Threshold=-500  SaturateOnIntegerOverflow=off  InputSameDT=off
  Throttle Saturation : Saturate  UpperLimit=MAX_TORQUE  LowerLimit=MIN_TORQUE
  second-order low-pass brake model1 : DiscreteTransferFcn  Commented=through  Numerator=DEND_B  Denominator=NUMD_B  SampleTime=ts
  second-order low-pass torque model : DiscreteTransferFcn  Commented=through  Numerator=DEND_T  Denominator=NUMD_T  SampleTime=ts
  torque_cm : Outport
  brake_cm : Outport  Port=2
  wires:
  Subsystem2/1(T_eng_cmd) -> second-order low-pass torque model/1
  acc_cmd/1 -> Subsystem2/1(acc_cmd)
  second-order low-pass brake model1/1 -> Brake Saturation/1
  Subsystem2/2(brake_cmd) -> second-order low-pass brake model1/1
  decc_cmd/1 -> Subsystem2/2(decc_cmd)
  second-order low-pass torque model/1 -> Throttle Saturation/1
  Throttle Saturation/1 -> Switch/2, Switch/1
  Switch/1 -> torque_cm/1
  Brake Saturation/1 -> Switch1/2, Switch1/3
  Switch1/1 -> brake_cm/1
  Constant/1 -> Switch/3, Switch1/1

== system IntModelY1/Controllers/Subsystem3/Subsystem2 ==
  acc_cmd : Inport
  Action Port : ActionPort  ActionPortLabel=case [ 1 ]:
  Brake Saturation : Saturate  UpperLimit=MAX_BRAKE  LowerLimit=MIN_BRAKE
  Constant : Constant  Value=0
  Gain : Gain  Commented=through  Gain=5
  Gain1 : Gain  Commented=through  Gain=5
  MATLAB Function : MATLAB Function  TreatAsAtomicUnit=on
  Subsystem2 : Subsystem
  Switch : Switch  Criteria=u2 > Threshold  Threshold=500  SaturateOnIntegerOverflow=off  InputSameDT=off
  Switch1 : Switch  Criteria=u2 > Threshold  Threshold=-500  SaturateOnIntegerOverflow=off  InputSameDT=off
  Throttle Saturation : Saturate  UpperLimit=MAX_TORQUE  LowerLimit=MIN_TORQUE
  second-order low-pass brake model1 : DiscreteTransferFcn  Commented=through  Numerator=DEND_B  Denominator=NUMD_B  SampleTime=ts
  second-order low-pass torque model : DiscreteTransferFcn  Commented=through  Numerator=DEND_T  Denominator=NUMD_T  SampleTime=ts
  torque_cm : Outport
  brake_cm : Outport  Port=2
  wires:
  second-order low-pass brake model1/1 -> Brake Saturation/1
  second-order low-pass torque model/1 -> Throttle Saturation/1
  Throttle Saturation/1 -> Switch/2, Switch/1
  Switch/1 -> torque_cm/1
  Brake Saturation/1 -> Switch1/2, Switch1/3
  Switch1/1 -> brake_cm/1
  Constant/1 -> Switch/3, Switch1/1
  acc_cmd/1 -> MATLAB Function/1(u)
  MATLAB Function/1(accel) -> Subsystem2/1(acc_cmd)
  MATLAB Function/2(decel) -> Subsystem2/2(decc_cmd)
  Subsystem2/1(T_eng_cmd) -> Gain/1
  Gain/1 -> second-order low-pass torque model/1
  Gain1/1 -> second-order low-pass brake model1/1
  Subsystem2/2(brake_cmd) -> Gain1/1
